simulink model "TCAS"  (R2020a)
settings: Solver=VariableStepAuto  StartTime=0.0  StopTime=100  RelTol=1e-3
values from neighbouring files (symbols this model uses):
  A_lqr = [A zeros(4, 1) ... (first row only)    [Model.m]
  aa0 = 2.52*(pi/180)    (= 0.0439822971503)    [const_atr72_3.m]
  aa_RMS = 5e-3    (= 0.005)    [const_atr72_3.m]
  B_lqr = [B ... (first row only)    [Model.m]
  C_lqr = eye(5)    [Model.m]
  D_lqr = zeros(5,2)    [Model.m]
  demax = +26*(pi/180)    (= 0.453785605519)    [const_atr72_3.m]
  demin = -22*(pi/180)    (= -0.383972435439)    [const_atr72_3.m]
  dtmax = 1    [const_atr72_3.m]
  dtmin = 0    [const_atr72_3.m]
  f_amostr = 40    [const_atr72_3.m]
  G0_inv = -([C_lqr(1,:);C_lqr(5,:)]*((A_lqr-B_lqr*Klqr)^(-1))*B_lqr*kuh)^(-1)    [Model.m]
  h = 7620    [const_atr72_3.m]
  Klqr = lqr(A_lqr, B_lqr, Q, R)    [Model.m]
  kuh = [Klqr(:,1),Klqr(:,5)]    [Model.m]
  raz_ang_RMS = 2e-3    (= 0.002)    [const_atr72_3.m]
  T_ang_aero = 0.01    [const_atr72_3.m]
  T_TAS = 0.1    [const_atr72_3.m]
  Tde = 0.1    [const_atr72_3.m]
  Teng = 0.80    (= 0.8)    [const_atr72_3.m]
  U0 = 275.3*0.514444444    (= 141.626555433)    [const_atr72_3.m]
  u_ref = 0    [Model.m]
  uW = 10    [Model.m]
  vmax_de = 60*(pi/180)    (= 1.0471975512)    [const_atr72_3.m]
  vmin_de = -60*(pi/180)    (= -1.0471975512)    [const_atr72_3.m]
undefined symbols (not defined in the file or in its folder): A_sensorh, B_sensorh, C_sensorh, caso, D_sensorh
libraries: simulink x12
settings Model: Creator=beapedroso  LastModifiedBy=tfesc
settings DataIOCC: ReturnWorkspaceOutputs=off
settings DebuggingCC: ArithmeticOperatorsInVariantConditions=warning
settings SFSimCC: SimUseLocalCustomCode=off  CustomCodeUndefinedFunction=UseInterfaceOnly
settings RTWCC: RTWUseLocalCustomCode=off

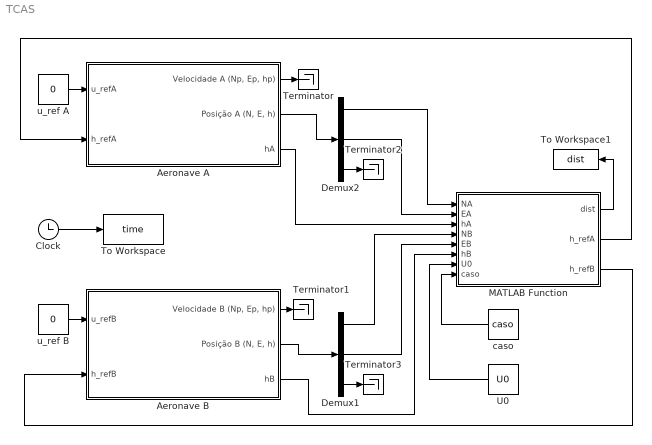
== system TCAS ==
  Aeronave A : Subsystem
  Aeronave B : Subsystem
  Clock : Clock
  Demux1 : Demux  Outputs=3
  Demux2 : Demux  Outputs=3
  MATLAB Function : MATLAB Function  TreatAsAtomicUnit=on
  Terminator{,1..3} (4 alike) : Terminator
  To Workspace : ToWorkspace  VariableName=time  SampleTime=1
  To Workspace1 : ToWorkspace  VariableName=dist  SaveFormat=Structure With Time  SampleTime=-1
  U0 : Constant  Value=U0
  caso : Constant  Value=caso
  u_ref A : Constant  Value=0
  u_ref B : Constant  Value=0
  wires:
  Aeronave A/1("Velocidade A (Np, Ep, hp)") -> Terminator/1
  Aeronave B/1("Velocidade B (Np, Ep, hp)") -> Terminator1/1
  Clock/1 -> To Workspace/1
  Aeronave B/2("Posição B (N, E, h)") -> Demux1/1
  Demux1/1 -> MATLAB Function/4(NB)
  Demux1/2 -> MATLAB Function/5(EB)
  U0/1 -> MATLAB Function/7(U0)
  Aeronave A/2("Posição A (N, E, h)") -> Demux2/1
  Demux2/1 -> MATLAB Function/1(NA)
  Demux2/2 -> MATLAB Function/2(EA)
  MATLAB Function/3(h_refB) -> Aeronave B/2(h_refB)
  MATLAB Function/2(h_refA) -> Aeronave A/2(h_refA)
  u_ref A/1 -> Aeronave A/1(u_refA)
  u_ref B/1 -> Aeronave B/1(u_refB)
  caso/1 -> MATLAB Function/8(caso)
  MATLAB Function/1(dist) -> To Workspace1/1
  Aeronave B/3(hB) -> MATLAB Function/6(hB)
  Aeronave A/3(hA) -> MATLAB Function/3(hA)
  Demux1/3 -> Terminator3/1
  Demux2/3 -> Terminator2/1

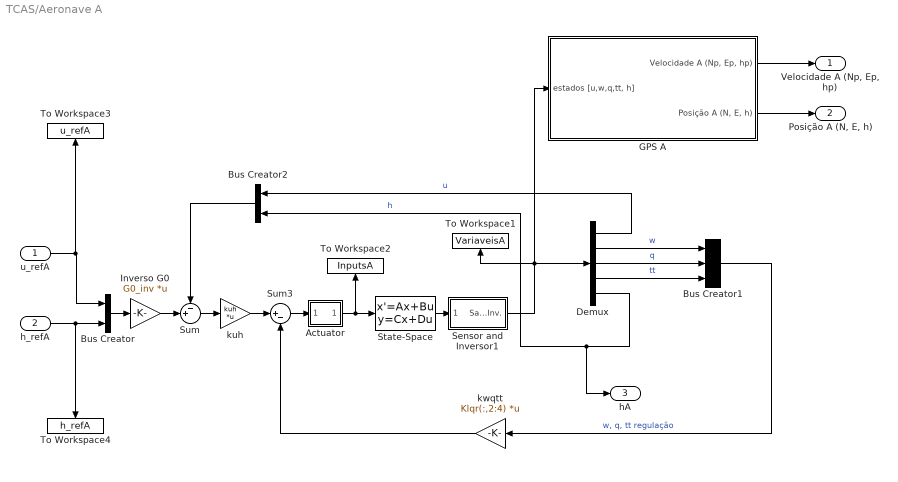
== system TCAS/Aeronave A ==
  u_refA : Inport
  h_refA : Inport  Port=2
  Actuator : Subsystem
  Bus Creator : BusCreator  Inputs=2
  Bus Creator1 : BusCreator  Inputs=3
  Bus Creator2 : BusCreator  Inputs=2
  Demux : Demux  Outputs=5
  GPS A : Subsystem
  Inverso G0 : Gain  Gain=G0_inv  Multiplication=Matrix(K*u)
  Sensor and Inversor1 : Subsystem
  State-Space : StateSpace  A=A_lqr  B=B_lqr  C=C_lqr  D=D_lqr  InitialCondition=[0,0,0,0,h]
  Sum : Sum  Inputs=-+|
  Sum3 : Sum  Inputs=|+-
  To Workspace1 : ToWorkspace  VariableName=VariaveisA  SaveFormat=Structure With Time  SampleTime=0.1
  To Workspace2 : ToWorkspace  VariableName=InputsA  SaveFormat=Structure With Time  SampleTime=0.1
  To Workspace3 : ToWorkspace  VariableName=u_refA  SaveFormat=Structure With Time  SampleTime=0.1
  To Workspace4 : ToWorkspace  VariableName=h_refA  SaveFormat=Structure With Time  SampleTime=0.1
  kuh : Gain  Gain=kuh  Multiplication=Matrix(K*u)
  kwqtt : Gain  Gain=Klqr(:,2:4)  Multiplication=Matrix(K*u)
  "Velocidade A (Np, Ep, hp)" : Outport  VectorParamsAs1DForOutWhenUnconnected=off
  "Posição A (N, E, h)" : Outport  Port=2  VectorParamsAs1DForOutWhenUnconnected=off
  hA : Outport  Port=3
  wires:
  GPS A/1("Velocidade A (Np, Ep, hp)") -> "Velocidade A (Np, Ep, hp)"/1
  GPS A/2("Posição A (N, E, h)") -> "Posição A (N, E, h)"/1
  kwqtt/1 -> Sum3/2
  Demux/3 -> Bus Creator1/2  "q"
  Demux/5 -> hA/1, Bus Creator2/2  "h"
  State-Space/1 -> Sensor and Inversor1/1(1)
  h_refA/1 -> Bus Creator/2, To Workspace4/1
  Bus Creator2/1 -> Sum/1
  Bus Creator1/1 -> kwqtt/1  "w, q, tt regulação"
  Inverso G0/1 -> Sum/2
  Demux/1 -> Bus Creator2/1  "u"
  Sum/1 -> kuh/1
  u_refA/1 -> Bus Creator/1, To Workspace3/1
  kuh/1 -> Sum3/1
  Demux/4 -> Bus Creator1/3  "tt"
  Bus Creator/1 -> Inverso G0/1
  Demux/2 -> Bus Creator1/1  "w"
  Sensor and Inversor1/1(Saída Inv.) -> To Workspace1/1, Demux/1, GPS A/1("estados [u,w,q,tt, h]")
  Sum3/1 -> Actuator/1(In1)
  Actuator/1(Out1) -> To Workspace2/1, State-Space/1

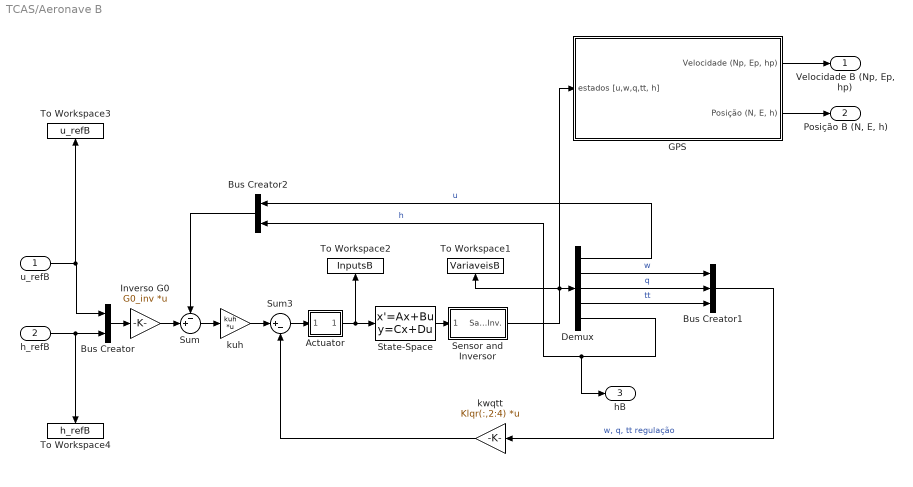
== system TCAS/Aeronave B ==
  u_refB : Inport
  h_refB : Inport  Port=2
  Actuator : Subsystem
  Bus Creator : BusCreator  Inputs=2
  Bus Creator1 : BusCreator  Inputs=3
  Bus Creator2 : BusCreator  Inputs=2
  Demux : Demux  Outputs=5
  GPS : Subsystem
  Inverso G0 : Gain  Gain=G0_inv  Multiplication=Matrix(K*u)
  Sensor and Inversor : Subsystem
  State-Space : StateSpace  A=A_lqr  B=B_lqr  C=C_lqr  D=D_lqr  InitialCondition=[0,0,0,0,h]
  Sum : Sum  Inputs=-+|
  Sum3 : Sum  Inputs=|+-
  To Workspace1 : ToWorkspace  VariableName=VariaveisB  SaveFormat=Structure With Time  SampleTime=0.1
  To Workspace2 : ToWorkspace  VariableName=InputsB  SaveFormat=Structure With Time  SampleTime=0.1
  To Workspace3 : ToWorkspace  VariableName=u_refB  SaveFormat=Structure With Time  SampleTime=0.1
  To Workspace4 : ToWorkspace  VariableName=h_refB  SaveFormat=Structure With Time  SampleTime=0.1
  kuh : Gain  Gain=kuh  Multiplication=Matrix(K*u)
  kwqtt : Gain  Gain=Klqr(:,2:4)  Multiplication=Matrix(K*u)
  "Velocidade B (Np, Ep, hp)" : Outport  VectorParamsAs1DForOutWhenUnconnected=off
  "Posição B (N, E, h)" : Outport  Port=2  VectorParamsAs1DForOutWhenUnconnected=off
  hB : Outport  Port=3
  wires:
  GPS/1("Velocidade (Np, Ep, hp)") -> "Velocidade B (Np, Ep, hp)"/1
  GPS/2("Posição (N, E, h)") -> "Posição B (N, E, h)"/1
  Demux/1 -> Bus Creator2/1  "u"
  h_refB/1 -> Bus Creator/2, To Workspace4/1
  Sum/1 -> kuh/1
  Demux/4 -> Bus Creator1/3  "tt"
  u_refB/1 -> Bus Creator/1, To Workspace3/1
  kwqtt/1 -> Sum3/2
  Bus Creator2/1 -> Sum/1
  Inverso G0/1 -> Sum/2
  Demux/3 -> Bus Creator1/2  "q"
  Demux/2 -> Bus Creator1/1  "w"
  Bus Creator1/1 -> kwqtt/1  "w, q, tt regulação"
  Bus Creator/1 -> Inverso G0/1
  kuh/1 -> Sum3/1
  State-Space/1 -> Sensor and Inversor/1(1)
  Sensor and Inversor/1(Saída Inv.) -> GPS/1("estados [u,w,q,tt, h]"), To Workspace1/1, Demux/1
  Sum3/1 -> Actuator/1(In1)
  Actuator/1(Out1) -> State-Space/1, To Workspace2/1
  Demux/5 -> hB/1, Bus Creator2/2  "h"

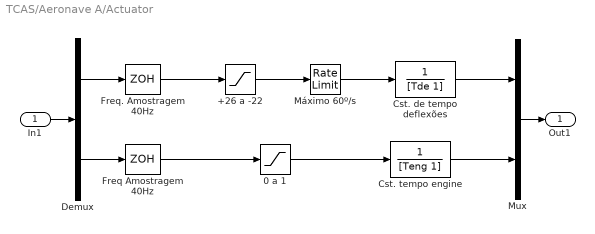
== system TCAS/Aeronave A/Actuator ==
  In1 : Inport
  +26 a -22 : Saturate  UpperLimit=demax  LowerLimit=demin
  0 a 1 : Saturate  UpperLimit=dtmax  LowerLimit=dtmin
  Cst. de tempo deflexões : TransferFcn  Denominator=[Tde 1]
  Cst. tempo engine : TransferFcn  Denominator=[Teng 1]
  Demux : Demux  Outputs=2
  Freq Amostragem 40Hz : ZeroOrderHold  SampleTime=1/f_amostr
  Freq. Amostragem 40Hz : ZeroOrderHold  SampleTime=1/f_amostr
  Mux : Mux  Inputs=2
  Máximo 60º/s : RateLimiter  RisingSlewLimit=vmax_de  FallingSlewLimit=vmin_de  SampleTimeMode=inherited  LinearizeAsGain=off
  Out1 : Outport
  wires:
  Freq. Amostragem 40Hz/1 -> +26 a -22/1
  Freq Amostragem 40Hz/1 -> 0 a 1/1
  +26 a -22/1 -> Máximo 60º/s/1
  Máximo 60º/s/1 -> Cst. de tempo deflexões/1
  0 a 1/1 -> Cst. tempo engine/1
  Demux/1 -> Freq. Amostragem 40Hz/1
  Mux/1 -> Out1/1
  In1/1 -> Demux/1
  Demux/2 -> Freq Amostragem 40Hz/1
  Cst. tempo engine/1 -> Mux/2
  Cst. de tempo deflexões/1 -> Mux/1

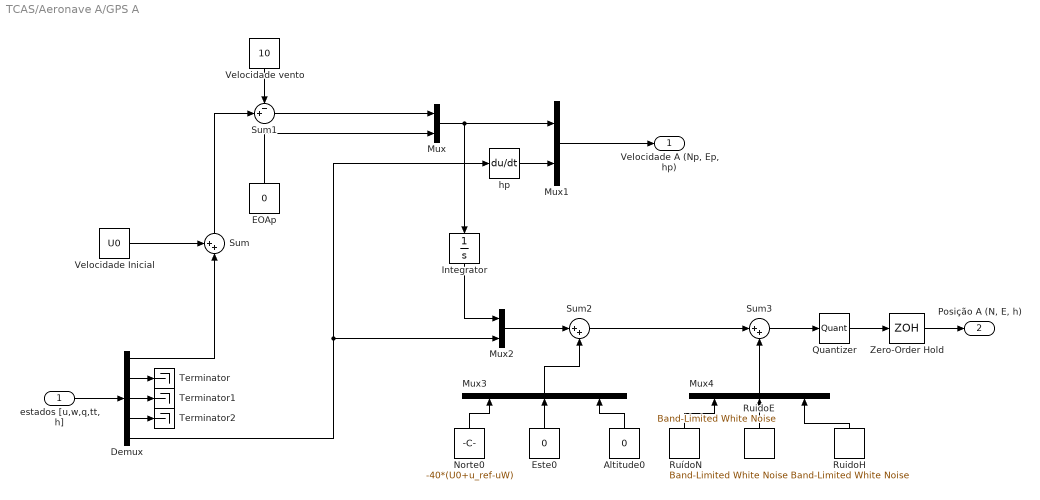
== system TCAS/Aeronave A/GPS A ==
  "estados [u,w,q,tt, h]" : Inport
  Altitude0 : Constant  Value=0
  Demux : Demux  Outputs=5
  EOAp : Constant  Value=0
  Este0 : Constant  Value=0
  Integrator : Integrator
  Mux : Mux  Inputs=2
  Mux1 : Mux  Inputs=2
  Mux2 : Mux  Inputs=2
  Mux3 : Mux  Inputs=3
  Mux4 : Mux  Inputs=3
  Norte0 : Constant  Value=-40*(U0+u_ref-uW)
  Quantizer : Quantizer
  RuidoE : simulink/Sources/Band-Limited White Noise  Cov=[0.1]  Ts=0.1  seed=[23341]
  RuidoH : simulink/Sources/Band-Limited White Noise  Cov=[0.1]  Ts=0.1  seed=[23341]
  RuídoN : simulink/Sources/Band-Limited White Noise  Cov=[0.1]  Ts=0.1  seed=[23341]
  Sum : Sum  Inputs=++|
  Sum1 : Sum  Inputs=-+|
  Sum2 : Sum  Inputs=|++
  Sum3 : Sum  Inputs=|++
  Terminator : Terminator
  Terminator1 : Terminator
  Terminator2 : Terminator
  "Velocidade Inicial " : Constant  Value=U0
  Velocidade vento : Constant  Value=10
  Zero-Order Hold : ZeroOrderHold  SampleTime=0.1
  "hp " : Derivative
  "Velocidade A (Np, Ep, hp)" : Outport  VectorParamsAs1DForOutWhenUnconnected=off
  "Posição A (N, E, h)" : Outport  Port=2  VectorParamsAs1DForOutWhenUnconnected=off
  wires:
  Demux/3 -> Terminator1/1
  "Velocidade Inicial "/1 -> Sum/1
  Velocidade vento/1 -> Sum1/1
  Integrator/1 -> Mux2/1
  "hp "/1 -> Mux1/2
  Mux3/1 -> Sum2/2
  Este0/1 -> Mux3/2
  Norte0/1 -> Mux3/1
  Mux2/1 -> Sum2/1
  Demux/1 -> Sum/2
  Altitude0/1 -> Mux3/3
  Mux1/1 -> "Velocidade A (Np, Ep, hp)"/1
  Demux/4 -> Terminator2/1
  Demux/2 -> Terminator/1
  "estados [u,w,q,tt, h]"/1 -> Demux/1
  Demux/5 -> Mux2/2, "hp "/1
  Mux/1 -> Integrator/1, Mux1/1
  Sum1/1 -> Mux/1
  Sum/1 -> Sum1/2
  EOAp/1 -> Mux/2
  Mux4/1 -> Sum3/2
  RuídoN/1 -> Mux4/1
  Zero-Order Hold/1 -> "Posição A (N, E, h)"/1
  Sum2/1 -> Sum3/1
  RuidoH/1 -> Mux4/3
  RuidoE/1 -> Mux4/2
  Quantizer/1 -> Zero-Order Hold/1
  Sum3/1 -> Quantizer/1

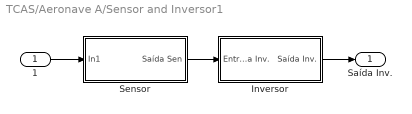
== system TCAS/Aeronave A/Sensor and Inversor1 ==
  1 : Inport
  Inversor : Subsystem
  Sensor : Subsystem
  Saída Inv. : Outport
  wires:
  1/1 -> Sensor/1(In1)
  Sensor/1(Saída Sen) -> Inversor/1(Entrada Inv.)
  Inversor/1(Saída Inv.) -> Saída Inv./1

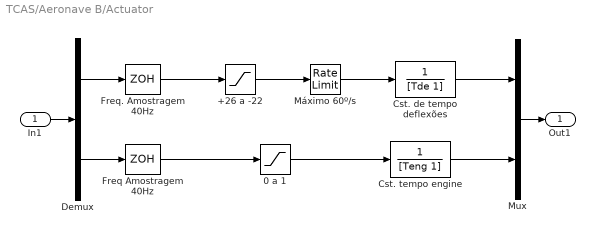
== system TCAS/Aeronave B/Actuator ==
  In1 : Inport
  +26 a -22 : Saturate  UpperLimit=demax  LowerLimit=demin
  0 a 1 : Saturate  UpperLimit=dtmax  LowerLimit=dtmin
  Cst. de tempo deflexões : TransferFcn  Denominator=[Tde 1]
  Cst. tempo engine : TransferFcn  Denominator=[Teng 1]
  Demux : Demux  Outputs=2
  Freq Amostragem 40Hz : ZeroOrderHold  SampleTime=1/f_amostr
  Freq. Amostragem 40Hz : ZeroOrderHold  SampleTime=1/f_amostr
  Mux : Mux  Inputs=2
  Máximo 60º/s : RateLimiter  RisingSlewLimit=vmax_de  FallingSlewLimit=vmin_de  SampleTimeMode=inherited  LinearizeAsGain=off
  Out1 : Outport
  wires:
  Freq. Amostragem 40Hz/1 -> +26 a -22/1
  Freq Amostragem 40Hz/1 -> 0 a 1/1
  +26 a -22/1 -> Máximo 60º/s/1
  Máximo 60º/s/1 -> Cst. de tempo deflexões/1
  0 a 1/1 -> Cst. tempo engine/1
  Demux/1 -> Freq. Amostragem 40Hz/1
  Mux/1 -> Out1/1
  In1/1 -> Demux/1
  Demux/2 -> Freq Amostragem 40Hz/1
  Cst. tempo engine/1 -> Mux/2
  Cst. de tempo deflexões/1 -> Mux/1

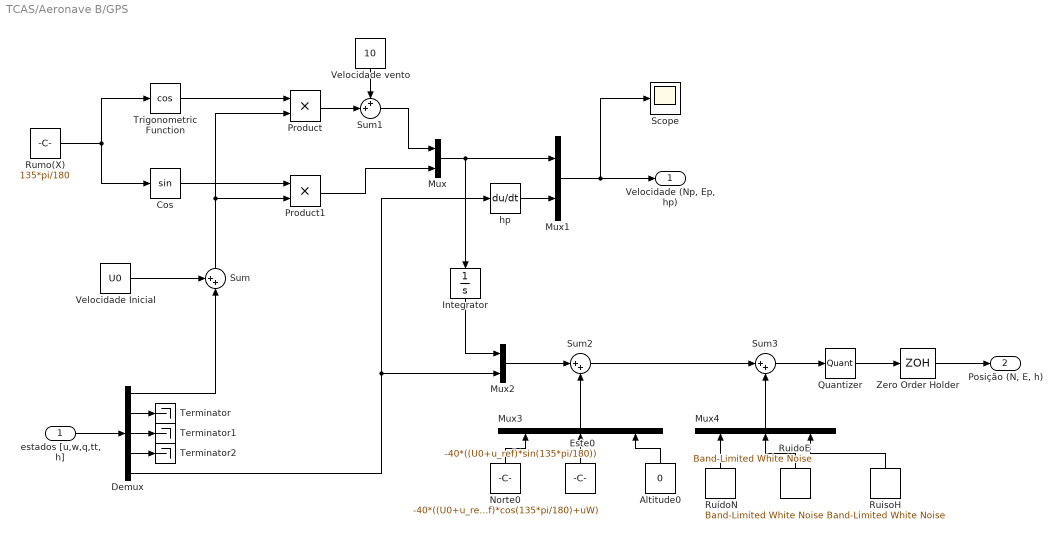
== system TCAS/Aeronave B/GPS ==
  "estados [u,w,q,tt, h]" : Inport
  Altitude0 : Constant  Value=0
  Cos : Trigonometry
  Demux : Demux  Outputs=5
  Este0 : Constant  Value=-40*((U0+u_ref)*sin(135*pi/180))
  Integrator : Integrator
  Mux : Mux  Inputs=2
  Mux1 : Mux  Inputs=2
  Mux2 : Mux  Inputs=2
  Mux3 : Mux  Inputs=3
  Mux4 : Mux  Inputs=3
  Norte0 : Constant  Value=-40*((U0+u_ref)*cos(135*pi/180)+uW)
  Product : Product
  Product1 : Product
  Quantizer : Quantizer
  RuidoE : simulink/Sources/Band-Limited White Noise  Cov=[0.1]  Ts=0.1  seed=[23341]
  RuisoH : simulink/Sources/Band-Limited White Noise  Cov=[0.1]  Ts=0.1  seed=[23341]
  "Rumo(X) " : Constant  Value=135*pi/180
  RuídoN : simulink/Sources/Band-Limited White Noise  Cov=[0.1]  Ts=0.1  seed=[23341]
  Scope : Scope
  Sum : Sum  Inputs=++|
  Sum1 : Sum  Inputs=++|
  Sum2 : Sum  Inputs=|++
  Sum3 : Sum  Inputs=|++
  Terminator : Terminator
  Terminator1 : Terminator
  Terminator2 : Terminator
  Trigonometric Function : Trigonometry  Operator=cos
  "Velocidade Inicial " : Constant  Value=U0
  Velocidade vento : Constant  Value=10
  Zero Order Holder : ZeroOrderHold  SampleTime=0.1
  "hp " : Derivative
  "Velocidade (Np, Ep, hp)" : Outport  VectorParamsAs1DForOutWhenUnconnected=off
  "Posição (N, E, h)" : Outport  Port=2  VectorParamsAs1DForOutWhenUnconnected=off
  wires:
  Demux/3 -> Terminator1/1
  Cos/1 -> Product1/1
  "Velocidade Inicial "/1 -> Sum/1
  Velocidade vento/1 -> Sum1/1
  Sum/1 -> Product1/2, Product/2
  Integrator/1 -> Mux2/1
  "hp "/1 -> Mux1/2
  Mux3/1 -> Sum2/2
  Este0/1 -> Mux3/2
  Norte0/1 -> Mux3/1
  "Rumo(X) "/1 -> Trigonometric Function/1, Cos/1
  Product1/1 -> Mux/2
  Mux2/1 -> Sum2/1
  Demux/1 -> Sum/2
  Altitude0/1 -> Mux3/3
  Mux1/1 -> Scope/1, "Velocidade (Np, Ep, hp)"/1
  Demux/4 -> Terminator2/1
  Demux/2 -> Terminator/1
  Trigonometric Function/1 -> Product/1
  "estados [u,w,q,tt, h]"/1 -> Demux/1
  Demux/5 -> Mux2/2, "hp "/1
  Mux/1 -> Integrator/1, Mux1/1
  Sum1/1 -> Mux/1
  Product/1 -> Sum1/2
  Sum2/1 -> Sum3/1
  RuídoN/1 -> Mux4/1
  RuidoE/1 -> Mux4/2
  RuisoH/1 -> Mux4/3
  Quantizer/1 -> Zero Order Holder/1
  Zero Order Holder/1 -> "Posição (N, E, h)"/1
  Mux4/1 -> Sum3/2
  Sum3/1 -> Quantizer/1

== system TCAS/Aeronave B/Sensor and Inversor ==
  1 : Inport
  Inversor : Subsystem
  Sensor : Subsystem
  Saída Inv. : Outport
  wires:
  1/1 -> Sensor/1(In1)
  Sensor/1(Saída Sen) -> Inversor/1(Entrada Inv.)
  Inversor/1(Saída Inv.) -> Saída Inv./1

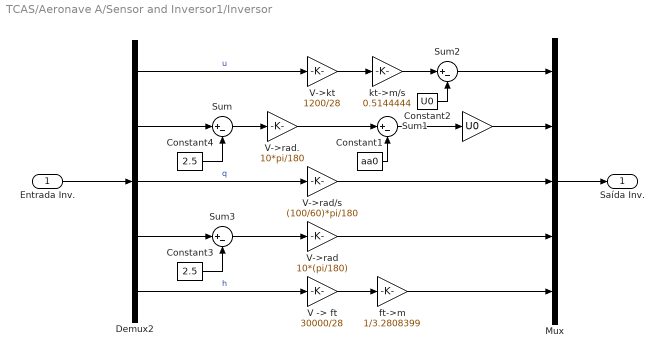
== system TCAS/Aeronave A/Sensor and Inversor1/Inversor ==
  Entrada Inv. : Inport
  " " : Gain  Gain=U0
  Constant1 : Constant  Value=aa0
  Constant2 : Constant  Value=U0
  Constant3 : Constant  Value=2.5
  Constant4 : Constant  Value=2.5
  Demux2 : Demux  Outputs=5
  Mux : Mux  Inputs=5
  Sum{,1..3} (4 alike) : Sum  Inputs=|+-
  "V -> ft" : Gain  Gain=30000/28
  V->kt : Gain  Gain=1200/28
  V->rad : Gain  Gain=10*(pi/180)
  V->rad. : Gain  Gain=10*pi/180
  V->rad/s : Gain  Gain=(100/60)*pi/180
  ft->m : Gain  Gain=1/3.2808399
  kt->m/s : Gain  Gain=0.5144444
  Saída Inv. : Outport  VectorParamsAs1DForOutWhenUnconnected=off
  wires:
  Constant1/1 -> Sum1/2
  Demux2/3 -> V->rad/s/1  "q"
  V->rad/s/1 -> Mux/3
  Demux2/1 -> V->kt/1  "u"
  Sum2/1 -> Mux/1
  Mux/1 -> Saída Inv./1
  Entrada Inv./1 -> Demux2/1
  V->kt/1 -> kt->m/s/1
  Constant2/1 -> Sum2/2
  V->rad./1 -> Sum1/1
  Sum1/1 -> " "/1
  " "/1 -> Mux/2
  Constant4/1 -> Sum/2
  Demux2/2 -> Sum/1
  Sum/1 -> V->rad./1
  kt->m/s/1 -> Sum2/1
  "V -> ft"/1 -> ft->m/1
  V->rad/1 -> Mux/4
  Demux2/4 -> Sum3/1
  Constant3/1 -> Sum3/2
  Sum3/1 -> V->rad/1
  Demux2/5 -> "V -> ft"/1  "h"
  ft->m/1 -> Mux/5

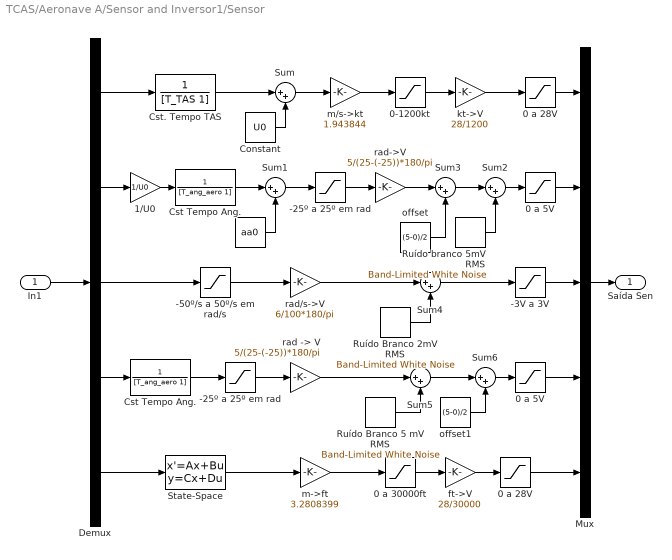
== system TCAS/Aeronave A/Sensor and Inversor1/Sensor ==
  In1 : Inport
  " " : Constant  Value=aa0
  -25º a 25º em rad : Saturate  UpperLimit=25*(pi/180)  LowerLimit=-25*(pi/180)
  "-25º a 25º em rad " : Saturate  UpperLimit=25*(pi/180)  LowerLimit=-25*(pi/180)
  -3V a 3V : Saturate  UpperLimit=3  LowerLimit=-3
  -50º/s a 50º/s em rad/s : Saturate  UpperLimit=50*(pi/180)  LowerLimit=-50*(pi/180)
  0 a 28V : Saturate  UpperLimit=28  LowerLimit=0
  "0 a 28V " : Saturate  UpperLimit=28  LowerLimit=-1
  0 a 30000ft : Saturate  UpperLimit=30000  LowerLimit=0
  0 a 5V : Saturate  UpperLimit=5  LowerLimit=0
  "0 a 5V " : Saturate  UpperLimit=5  LowerLimit=-5
  0-1200kt : Saturate  UpperLimit=1200  LowerLimit=0
  1/U0 : Gain  Gain=1/U0
  Constant : Constant  Value=U0
  Cst Tempo Ang. : TransferFcn  Denominator=[T_ang_aero 1]
  Cst Tempo Ang. : TransferFcn  Denominator=[T_ang_aero 1]
  "Cst. Tempo TAS " : TransferFcn  Denominator=[T_TAS 1]
  Demux : Demux  Outputs=5
  Mux : Mux  Inputs=5
  Ruído Branco 2mV RMS : simulink/Sources/Band-Limited White Noise  Cov=raz_ang_RMS^2/f_amostr  Ts=1/f_amostr  seed=[23356]
  Ruído Branco 5 mV RMS : simulink/Sources/Band-Limited White Noise  Cov=[aa_RMS^2/f_amostr]  Ts=1/f_amostr  seed=[23341]
  Ruído branco 5mV RMS : simulink/Sources/Band-Limited White Noise  Cov=[aa_RMS^2/f_amostr]  Ts=1/f_amostr  seed=[23341]
  State-Space : StateSpace  A=A_sensorh  B=B_sensorh  C=C_sensorh  D=D_sensorh  InitialCondition=762
  Sum{,1..6} (7 alike) : Sum  Inputs=|++
  ft->V : Gain  Gain=28/30000
  kt->V : Gain  Gain=28/1200
  m->ft : Gain  Gain=3.2808399
  m/s->kt : Gain  Gain=1.943844
  offset : Constant  Value=(5-0)/2
  offset1 : Constant  Value=(5-0)/2
  "rad -> V" : Gain  Gain=5/(25-(-25))*180/pi
  rad->V : Gain  Gain=5/(25-(-25))*180/pi
  rad/s->V : Gain  Gain=6/100*180/pi
  Saída Sen : Outport
  wires:
  In1/1 -> Demux/1
  Mux/1 -> Saída Sen/1
  Demux/1 -> "Cst. Tempo TAS "/1
  "Cst. Tempo TAS "/1 -> Sum/1
  Sum/1 -> m/s->kt/1
  Constant/1 -> Sum/2
  m/s->kt/1 -> 0-1200kt/1
  0-1200kt/1 -> kt->V/1
  Demux/2 -> 1/U0/1
  1/U0/1 -> Cst Tempo Ang./1
  Cst Tempo Ang./1 -> Sum1/1
  " "/1 -> Sum1/2
  Sum1/1 -> -25º a 25º em rad/1
  -25º a 25º em rad/1 -> rad->V/1
  Ruído branco 5mV RMS/1 -> Sum2/2
  Sum2/1 -> 0 a 5V/1
  Demux/3 -> -50º/s a 50º/s em rad/s/1
  -50º/s a 50º/s em rad/s/1 -> rad/s->V/1
  Ruído Branco 2mV RMS/1 -> Sum4/2
  rad/s->V/1 -> Sum4/1
  "-25º a 25º em rad "/1 -> "rad -> V"/1
  Ruído Branco 5 mV RMS/1 -> Sum5/2
  "rad -> V"/1 -> Sum5/1
  0 a 30000ft/1 -> ft->V/1
  Sum3/1 -> Sum2/1
  rad->V/1 -> Sum3/1
  offset/1 -> Sum3/2
  0 a 5V/1 -> Mux/2
  kt->V/1 -> 0 a 28V/1
  Sum4/1 -> -3V a 3V/1
  0 a 28V/1 -> Mux/1
  -3V a 3V/1 -> Mux/3
  "0 a 5V "/1 -> Mux/4
  Sum5/1 -> Sum6/1
  offset1/1 -> Sum6/2
  Sum6/1 -> "0 a 5V "/1
  Cst Tempo Ang./1 -> "-25º a 25º em rad "/1
  Demux/4 -> Cst Tempo Ang./1
  m->ft/1 -> 0 a 30000ft/1
  ft->V/1 -> "0 a 28V "/1
  "0 a 28V "/1 -> Mux/5
  Demux/5 -> State-Space/1
  State-Space/1 -> m->ft/1

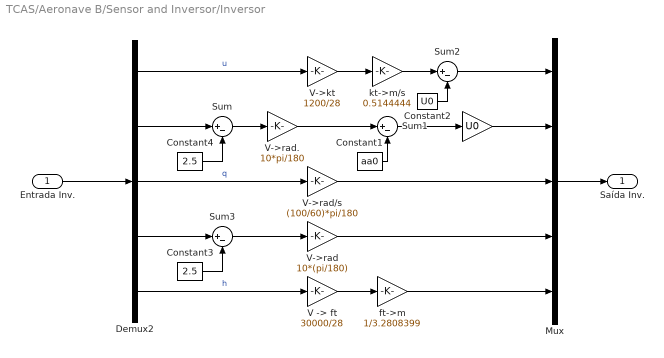
== system TCAS/Aeronave B/Sensor and Inversor/Inversor ==
  Entrada Inv. : Inport
  " " : Gain  Gain=U0
  Constant1 : Constant  Value=aa0
  Constant2 : Constant  Value=U0
  Constant3 : Constant  Value=2.5
  Constant4 : Constant  Value=2.5
  Demux2 : Demux  Outputs=5
  Mux : Mux  Inputs=5
  Sum{,1..3} (4 alike) : Sum  Inputs=|+-
  "V -> ft" : Gain  Gain=30000/28
  V->kt : Gain  Gain=1200/28
  V->rad : Gain  Gain=10*(pi/180)
  V->rad. : Gain  Gain=10*pi/180
  V->rad/s : Gain  Gain=(100/60)*pi/180
  ft->m : Gain  Gain=1/3.2808399
  kt->m/s : Gain  Gain=0.5144444
  Saída Inv. : Outport  VectorParamsAs1DForOutWhenUnconnected=off
  wires:
  Constant1/1 -> Sum1/2
  Demux2/3 -> V->rad/s/1  "q"
  V->rad/s/1 -> Mux/3
  Demux2/1 -> V->kt/1  "u"
  Sum2/1 -> Mux/1
  Mux/1 -> Saída Inv./1
  Entrada Inv./1 -> Demux2/1
  V->kt/1 -> kt->m/s/1
  Constant2/1 -> Sum2/2
  V->rad./1 -> Sum1/1
  Sum1/1 -> " "/1
  " "/1 -> Mux/2
  Constant4/1 -> Sum/2
  Demux2/2 -> Sum/1
  Sum/1 -> V->rad./1
  kt->m/s/1 -> Sum2/1
  "V -> ft"/1 -> ft->m/1
  V->rad/1 -> Mux/4
  Demux2/4 -> Sum3/1
  Constant3/1 -> Sum3/2
  Sum3/1 -> V->rad/1
  Demux2/5 -> "V -> ft"/1  "h"
  ft->m/1 -> Mux/5

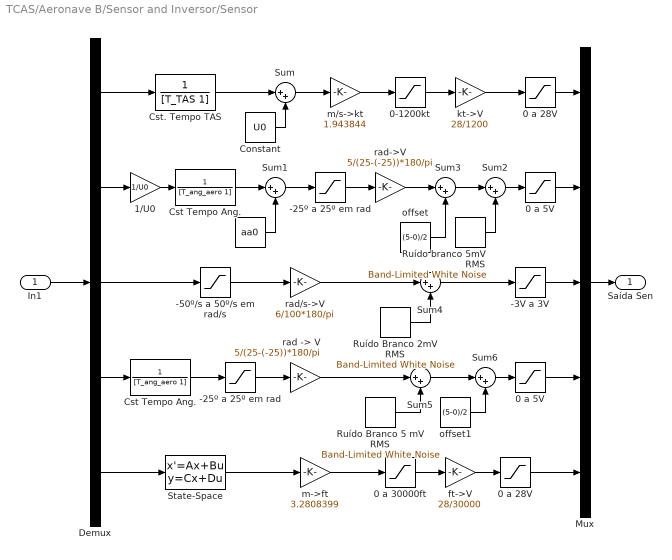
== system TCAS/Aeronave B/Sensor and Inversor/Sensor ==
  In1 : Inport
  " " : Constant  Value=aa0
  -25º a 25º em rad : Saturate  UpperLimit=25*(pi/180)  LowerLimit=-25*(pi/180)
  "-25º a 25º em rad " : Saturate  UpperLimit=25*(pi/180)  LowerLimit=-25*(pi/180)
  -3V a 3V : Saturate  UpperLimit=3  LowerLimit=-3
  -50º/s a 50º/s em rad/s : Saturate  UpperLimit=50*(pi/180)  LowerLimit=-50*(pi/180)
  0 a 28V : Saturate  UpperLimit=28  LowerLimit=0
  "0 a 28V " : Saturate  UpperLimit=28  LowerLimit=-1
  0 a 30000ft : Saturate  UpperLimit=30000  LowerLimit=0
  0 a 5V : Saturate  UpperLimit=5  LowerLimit=0
  "0 a 5V " : Saturate  UpperLimit=5  LowerLimit=-5
  0-1200kt : Saturate  UpperLimit=1200  LowerLimit=0
  1/U0 : Gain  Gain=1/U0
  Constant : Constant  Value=U0
  Cst Tempo Ang. : TransferFcn  Denominator=[T_ang_aero 1]
  Cst Tempo Ang. : TransferFcn  Denominator=[T_ang_aero 1]
  "Cst. Tempo TAS " : TransferFcn  Denominator=[T_TAS 1]
  Demux : Demux  Outputs=5
  Mux : Mux  Inputs=5
  Ruído Branco 2mV RMS : simulink/Sources/Band-Limited White Noise  Cov=raz_ang_RMS^2/f_amostr  Ts=1/f_amostr  seed=[23356]
  Ruído Branco 5 mV RMS : simulink/Sources/Band-Limited White Noise  Cov=[aa_RMS^2/f_amostr]  Ts=1/f_amostr  seed=[23341]
  Ruído branco 5mV RMS : simulink/Sources/Band-Limited White Noise  Cov=[aa_RMS^2/f_amostr]  Ts=1/f_amostr  seed=[23341]
  State-Space : StateSpace  A=A_sensorh  B=B_sensorh  C=C_sensorh  D=D_sensorh  InitialCondition=762
  Sum{,1..6} (7 alike) : Sum  Inputs=|++
  ft->V : Gain  Gain=28/30000
  kt->V : Gain  Gain=28/1200
  m->ft : Gain  Gain=3.2808399
  m/s->kt : Gain  Gain=1.943844
  offset : Constant  Value=(5-0)/2
  offset1 : Constant  Value=(5-0)/2
  "rad -> V" : Gain  Gain=5/(25-(-25))*180/pi
  rad->V : Gain  Gain=5/(25-(-25))*180/pi
  rad/s->V : Gain  Gain=6/100*180/pi
  Saída Sen : Outport
  wires:
  In1/1 -> Demux/1
  Mux/1 -> Saída Sen/1
  Demux/1 -> "Cst. Tempo TAS "/1
  "Cst. Tempo TAS "/1 -> Sum/1
  Sum/1 -> m/s->kt/1
  Constant/1 -> Sum/2
  m/s->kt/1 -> 0-1200kt/1
  0-1200kt/1 -> kt->V/1
  Demux/2 -> 1/U0/1
  1/U0/1 -> Cst Tempo Ang./1
  Cst Tempo Ang./1 -> Sum1/1
  " "/1 -> Sum1/2
  Sum1/1 -> -25º a 25º em rad/1
  -25º a 25º em rad/1 -> rad->V/1
  Ruído branco 5mV RMS/1 -> Sum2/2
  Sum2/1 -> 0 a 5V/1
  Demux/3 -> -50º/s a 50º/s em rad/s/1
  -50º/s a 50º/s em rad/s/1 -> rad/s->V/1
  Ruído Branco 2mV RMS/1 -> Sum4/2
  rad/s->V/1 -> Sum4/1
  "-25º a 25º em rad "/1 -> "rad -> V"/1
  Ruído Branco 5 mV RMS/1 -> Sum5/2
  "rad -> V"/1 -> Sum5/1
  0 a 30000ft/1 -> ft->V/1
  Sum3/1 -> Sum2/1
  rad->V/1 -> Sum3/1
  offset/1 -> Sum3/2
  0 a 5V/1 -> Mux/2
  kt->V/1 -> 0 a 28V/1
  Sum4/1 -> -3V a 3V/1
  0 a 28V/1 -> Mux/1
  -3V a 3V/1 -> Mux/3
  "0 a 5V "/1 -> Mux/4
  Sum5/1 -> Sum6/1
  offset1/1 -> Sum6/2
  Sum6/1 -> "0 a 5V "/1
  Cst Tempo Ang./1 -> "-25º a 25º em rad "/1
  Demux/4 -> Cst Tempo Ang./1
  m->ft/1 -> 0 a 30000ft/1
  ft->V/1 -> "0 a 28V "/1
  "0 a 28V "/1 -> Mux/5
  Demux/5 -> State-Space/1
  State-Space/1 -> m->ft/1

== matlab function TCAS/MATLAB Function ==
  data: NA input; dist output; EA input; hA input; NB input; EB input; hB input; U0 input; h_refA output; h_refB output; caso input
function [dist, h_refA, h_refB] = TCAS(NA,EA,hA,NB,EB,hB,U0,caso)

uW=10; %velocidade vento N-S
u_ref=0;
tt0=0.0440;

NOB25=25*((U0+u_ref)*sin(135*pi/180)+uW);
EOB25=25*((U0+u_ref)*cos(135*pi/180));

NOA25=-25*(U0+u_ref-uW);
EOA25=0;

h_inicial = 7620;
hB25=h_inicial;
hA25=h_inicial;

dist25=sqrt((NOB25-NOA25)^2+(EOB25-EOA25)^2+(hB25-hA25)^2);


dist=sqrt((NB-NA)^2+(EB-EA)^2+(hB-hA)^2);

%Caso 1 - Aeronave A altera trajetória
%Caso 2 - Ambas as aeronaves alteram a trajetória


if dist < dist25
     if caso == 0
        h_refA = h_inicial;
        h_refB = h_inicial;
     elseif caso == 1
        h_refA = h_inicial+180;
        h_refB = h_inicial;
     else
        h_refA = h_inicial+90;
        h_refB = h_inicial-90; 
    end
else
    h_refA = h_inicial;
    h_refB = h_inicial;   
end

end
